simulink subsystem "PvtSubSys_LATC"  (R2020b)
settings: Solver=VariableStepAuto  StartTime=0.0  StopTime=10.0  RelTol=1e-3
values from neighbouring files (symbols this model uses):
  P_Global_CharSpd_ms : value not decoded    [PubParsGlobal.sldd]
  P_Global_SteeringAngleRatio : value not decoded    [PubParsGlobal.sldd]
  P_Global_WheelBase_m : value not decoded    [PubParsGlobal.sldd]
  P_LCS_A0_Limit = 0.25    [LATC.sldd]    (also in LCS_v05.sldd)
  P_LCS_A1_Limit = 0.002    [LATC.sldd]    (also in LCS_v05.sldd)
  P_LCS_communicationTest = 1.0    [LATC.sldd]    (also in LCS_v05.sldd)
  P_LCS_Current_Offset_Test_SW = 0.0    [LATC.sldd]
  P_LCS_Current_Offset_Test_Value = 0.0    [LATC.sldd]
  P_LCS_Curvature_bp : value not decoded    [LATC.sldd]
  P_LCS_CycleTime = 0.4 0.4 0.4 0.4 0.4 0.4 0.4 0.4 0.4 0.6 0.6 0.6 0.6 0.6 0.6 0.6 0.4 0.4 0.4 0.4 0.4 0.4 0.4 0.4 0.4 0.6 0.6 0.6 0.6 0.6 0.6 0.6 0.4 0.4 0.4 0.4 0.4 0.4 0.4 0.4 0.4 0.6 0.6 0.6 0.6 0.6 0.6 0.6 0.4 0.4 0.4 0.4 0.4 0.4 0.4 0.4 0.4 0.6 0.6 0.6 0.6 0.6 0.6 0.6 0.4 0.4 0.4 0.4 0.4 0.4 0.4 0.4 0.4 0.6 0.6 0.6 0.6 0.6 0.6 0.6 0.4 0.4 0.4 0.4 0.4 0.4 0.4 0.4 0.4 0.6 0.6 0.6 0.6 0.6 0.6 0.6 0.4 0.4 0.4 0.4    [LATC.sldd]
  P_LCS_ESS_AngleSlope_Limit = 2.9    [LATC.sldd]    (also in LCS_v05.sldd)
  P_LCS_IN_Offset_Test_SW = 0.0    [LATC.sldd]    (also in LCS_v05.sldd)
  P_LCS_IN_Offset_Test_Value = 0.0    [LATC.sldd]    (also in LCS_v05.sldd)
  P_LCS_LATC_CurOffsetVehicleSpdLimitValue_degs = 7.0    [LATC.sldd]
  P_LCS_LATC_Du_Max = 20.0    [LATC.sldd]
  P_LCS_LATC_ELKAngleSlope_ratio : value not decoded    [LATC.sldd]
  P_LCS_LATC_ELKMaxLatAcc_ms2 : value not decoded    [LATC.sldd]
  P_LCS_LATC_ESSAngleSlope_ratio : value not decoded    [LATC.sldd]
  P_LCS_LATC_ESSMaxLatAcc_ms2 : value not decoded    [LATC.sldd]
  P_LCS_LATC_LCAngleSlope_ratio : value not decoded    [LATC.sldd]
  P_LCS_LATC_LCCancleMaxLatAcc_ms2 : value not decoded    [LATC.sldd]
  P_LCS_LATC_LCEcoAngleSlope_ratio : value not decoded    [LATC.sldd]
  P_LCS_LATC_LCEcoMaxLatAcc_ms2 : value not decoded    [LATC.sldd]
  P_LCS_LATC_LCKAngleSlope_ratio : value not decoded    [LATC.sldd]
  P_LCS_LATC_LCKIEAngleSlope_ratio : value not decoded    [LATC.sldd]
  P_LCS_LATC_LCKIEMaxLatAcc_ms2 : value not decoded    [LATC.sldd]
  P_LCS_LATC_LCKMaxLatAcc_ms2 : value not decoded    [LATC.sldd]
  P_LCS_LATC_LCNormalAngleSlope_ratio : value not decoded    [LATC.sldd]
  P_LCS_LATC_LCNormalMaxLatAcc_ms2 : value not decoded    [LATC.sldd]
  P_LCS_LATC_LCSportAngleSlope_ratio : value not decoded    [LATC.sldd]
  P_LCS_LATC_LCSportMaxLatAcc_ms2 : value not decoded    [LATC.sldd]
  P_LCS_LATC_LKAAngleSlope_ratio : value not decoded    [LATC.sldd]
  P_LCS_LATC_LKAMaxLatAcc_ms2 : value not decoded    [LATC.sldd]
  P_LCS_LATC_MatrixQ1_st = 0.8 0.8 1.2 1.4 1.4 1.4 2.0 2.2 2.2 2.2 2.2 2.2 2.2 2.2 2.2 2.2 0.8 0.8 1.2 1.4 1.4 1.4 2.0 2.2 2.2 2.2 2.2 2.2 2.2 2.2 2.2 2.2 0.8 0.8 1.2 1.4 1.4 1.4 2.0 2.2 2.2 2.2 2.2 2.2 2.2 2.2 2.2 2.2 0.8 0.8 1.2 1.4 1.4 1.4 2.0 2.2 2.2 2.2 2.2 2.2 2.2 2.2 2.2 2.2 0.8 0.8 1.2 1.4 1.4 1.4 2.0 2.2 2.2 2.2 2.2 2.2 2.2 2.2 2.2 2.2 0.8 0.8 1.2 1.4 1.4 1.4 2.0 2.2 2.2 2.2 2.2 2.2 2.2 2.2 2.2 2.2 0.8 0.8 1.2 1.4    [LATC.sldd]
  P_LCS_LATC_MatrixQ3_st = 20.0 20.0 20.0 20.0 20.0 15.0 15.0 15.0 15.0 15.0 15.0 15.0 15.0 13.0 13.0 13.0 20.0 20.0 20.0 20.0 20.0 15.0 15.0 15.0 15.0 15.0 15.0 15.0 15.0 13.0 13.0 13.0 20.0 20.0 20.0 20.0 20.0 15.0 15.0 15.0 15.0 15.0 15.0 15.0 15.0 13.0 13.0 13.0 20.0 20.0 20.0 20.0 20.0 15.0 15.0 15.0 15.0 15.0 15.0 15.0 15.0 13.0 13.0 13.0 20.0 20.0 20.0 20.0 20.0 15.0 15.0 15.0 15.0 15.0 15.0 15.0 15.0 13.0 13.0 13.0    [LATC.sldd]
  P_LCS_LATC_MatrixR_st = 10.0 10.0 10.0 10.0 10.0 10.0 10.0 15.0 15.0 15.0 15.0 15.0 15.0 15.0 15.0 15.0 10.0 10.0 10.0 10.0 10.0 10.0 10.0 15.0 15.0 15.0 15.0 15.0 15.0 15.0 15.0 15.0 10.0 10.0 10.0 10.0 10.0 10.0 10.0 15.0 15.0 15.0 15.0 15.0 15.0 15.0 15.0 15.0 10.0 10.0 10.0 10.0 10.0 10.0 10.0 15.0 15.0 15.0 15.0 15.0 15.0 15.0 15.0 15.0 10.0 10.0 10.0 10.0 10.0 10.0 10.0 15.0 15.0 15.0 15.0 15.0 15.0 15.0 15.0 15.0    [LATC.sldd]
  P_LCS_LATC_Max_LatAcc = 4.0    [LATC.sldd]
  P_LCS_LATC_Max_Phi = 15.0    [LATC.sldd]
  P_LCS_LATC_Max_y = 0.5    [LATC.sldd]
  P_LCS_LATC_MPC_SW = 0.0    [LATC.sldd]
  P_LCS_LATC_PreView_SW = 1.0    [LATC.sldd]
  P_LCS_LATC_SoftConstWeight = 1.0    [LATC.sldd]
  P_LCS_LATC_StateActivAngleSlopeLimit_ratio : value not decoded    [LATC.sldd]
  P_LCS_LATC_StateActiveFlg_TabX_st : value not decoded    [LATC.sldd]
  P_LCS_LATC_StateActiveHoldTime_TabY_st : value not decoded    [LATC.sldd]
  P_LCS_LATC_StateHoldTime_st = 250.0    [LATC.sldd]
  P_LCS_LATC_TarAngleFliterWindowSize = 5.0    [LATC.sldd]
  P_LCS_LATC_TarAngleLP_Time = 0.02    [LATC.sldd]
  P_LCS_LATC_U_Max = 90.0    [LATC.sldd]
  P_LCS_LCK_AngleSlope_Limit = 1.4    [LATC.sldd]
  P_LCS_LineVaildSW = 0.0    [LATC.sldd]
  P_LCS_Lookahead_Distance : value not decoded    [LATC.sldd]
  P_LCS_Lookahead_DistanceFac : value not decoded    [LATC.sldd]
  P_LCS_PLAN_CurvePreView_s = 0.3    [LATC.sldd]
  P_LCS_PLAN_CurvePreview_TabX_m : value not decoded    [LATC.sldd]
  P_LCS_PLAN_CurvePreViewFilterTime_s = 0.1    [LATC.sldd]
  P_LCS_PLAN_ELKAyDtLimit_Tab_ms3 = 1.0 1.0 1.0 1.0 1.0 1.0 1.0 1.0 1.0 1.0 1.0 1.0 1.0 1.0 1.0 1.0 1.0 1.0 1.0 1.0 1.0 1.0 1.0 1.0 1.0 1.0 1.0 1.0 1.0 1.0 1.0 1.0 1.0 1.0 1.0 1.0 1.0 1.0 1.0 1.0 1.0 1.0 1.0 1.0 1.0 1.0 1.0 1.0 1.0 1.0 1.0 1.0 1.0 1.0 1.0 1.0 1.0 1.0 1.0 1.0 1.0 1.0 1.0 1.0 1.0 1.0 1.0 1.0 1.0 1.0 1.0 1.0 1.0 1.0 1.0 1.0 1.0 1.0 1.0 1.0 1.0 1.0 1.0 1.0 1.0 1.0 1.0 1.0 1.0 1.0 1.0 1.0 1.0 1.0 1.0 1.0 1.0 1.0 1.0 1.0    [LATC.sldd]
  P_LCS_PLAN_ESSAyDtLimit_Tab_ms3 = 1.0 1.0 1.0 1.0 1.0 1.0 1.0 1.0 1.0 1.0 1.0 1.0 1.0 1.0 1.0 1.0 1.0 1.0 1.0 1.0 1.0 1.0 1.0 1.0 1.0 1.0 1.0 1.0 1.0 1.0 1.0 1.0 1.0 1.0 1.0 1.0 1.0 1.0 1.0 1.0 1.0 1.0 1.0 1.0 1.0 1.0 1.0 1.0 1.0 1.0 1.0 1.0 1.0 1.0 1.0 1.0 1.0 1.0 1.0 1.0 1.0 1.0 1.0 1.0 1.0 1.0 1.0 1.0 1.0 1.0 1.0 1.0 1.0 1.0 1.0 1.0 1.0 1.0 1.0 1.0 1.0 1.0 1.0 1.0 1.0 1.0 1.0 1.0 1.0 1.0 1.0 1.0 1.0 1.0 1.0 1.0 1.0 1.0 1.0 1.0    [LATC.sldd]
  P_LCS_PLAN_LCCancleAyDtLimit_Tab_ms3 = 1.0 1.0 1.0 1.0 1.0 1.0 1.0 1.0 1.0 1.0 1.0 1.0 1.0 1.0 1.0 1.0 1.0 1.0 1.0 1.0 1.0 1.0 1.0 1.0 1.0 1.0 1.0 1.0 1.0 1.0 1.0 1.0 1.0 1.0 1.0 1.0 1.0 1.0 1.0 1.0 1.0 1.0 1.0 1.0 1.0 1.0 1.0 1.0 1.0 1.0 1.0 1.0 1.0 1.0 1.0 1.0 1.0 1.0 1.0 1.0 1.0 1.0 1.0 1.0 1.0 1.0 1.0 1.0 1.0 1.0 1.0 1.0 1.0 1.0 1.0 1.0 1.0 1.0 1.0 1.0 1.0 1.0 1.0 1.0 1.0 1.0 1.0 1.0 1.0 1.0 1.0 1.0 1.0 1.0 1.0 1.0 1.0 1.0 1.0 1.0    [LATC.sldd]
  P_LCS_PLAN_LCEcoAyDtLimit_Tab_ms3 = 1.0 1.0 1.0 1.0 1.0 1.0 1.0 1.0 1.0 1.0 1.0 1.0 1.0 1.0 1.0 1.0 1.0 1.0 1.0 1.0 1.0 1.0 1.0 1.0 1.0 1.0 1.0 1.0 1.0 1.0 1.0 1.0 1.0 1.0 1.0 1.0 1.0 1.0 1.0 1.0 1.0 1.0 1.0 1.0 1.0 1.0 1.0 1.0 1.0 1.0 1.0 1.0 1.0 1.0 1.0 1.0 1.0 1.0 1.0 1.0 1.0 1.0 1.0 1.0 1.0 1.0 1.0 1.0 1.0 1.0 1.0 1.0 1.0 1.0 1.0 1.0 1.0 1.0 1.0 1.0 1.0 1.0 1.0 1.0 1.0 1.0 1.0 1.0 1.0 1.0 1.0 1.0 1.0 1.0 1.0 1.0 1.0 1.0 1.0 1.0    [LATC.sldd]
  P_LCS_PLAN_LCKAyDtLimit_Tab_ms3 = 1.5 1.5 1.5 1.5 1.5 1.5 1.5 1.5 1.5 1.5 1.5 1.5 1.5 1.5 1.5 1.5 1.5 1.5 1.5 1.5 1.5 1.5 1.5 1.5 1.5 1.5 1.5 1.5 1.5 1.5 1.5 1.5 1.5 1.5 1.5 1.5 1.5 1.5 1.5 1.5 1.5 1.5 1.5 1.5 1.5 1.5 1.5 1.5 1.5 1.5 1.5 1.5 1.5 1.5 1.5 1.5 1.5 1.5 1.5 1.5 1.5 1.5 1.5 1.5 1.5 1.5 1.5 1.5 1.5 1.5 1.5 1.5 1.5 1.5 1.5 1.5 1.5 1.5 1.5 1.5 1.5 1.5 1.5 1.5 1.5 1.5 1.5 1.5 1.5 1.5 1.5 1.5 1.5 1.5 1.5 1.5 1.5 1.5 1.5 1.5    [LATC.sldd]
  P_LCS_PLAN_LCKIEAyDtLimit_Tab_ms3 = 1.0 1.0 1.0 1.0 1.0 1.0 1.0 1.0 1.0 1.0 1.0 1.0 1.0 1.0 1.0 1.0 1.0 1.0 1.0 1.0 1.0 1.0 1.0 1.0 1.0 1.0 1.0 1.0 1.0 1.0 1.0 1.0 1.0 1.0 1.0 1.0 1.0 1.0 1.0 1.0 1.0 1.0 1.0 1.0 1.0 1.0 1.0 1.0 1.0 1.0 1.0 1.0 1.0 1.0 1.0 1.0 1.0 1.0 1.0 1.0 1.0 1.0 1.0 1.0 1.0 1.0 1.0 1.0 1.0 1.0 1.0 1.0 1.0 1.0 1.0 1.0 1.0 1.0 1.0 1.0 1.0 1.0 1.0 1.0 1.0 1.0 1.0 1.0 1.0 1.0 1.0 1.0 1.0 1.0 1.0 1.0 1.0 1.0 1.0 1.0    [LATC.sldd]
  P_LCS_PLAN_LCNormalAyDtLimit_Tab_ms3 = 1.0 1.0 1.0 1.0 1.0 1.0 1.0 1.0 1.0 1.0 1.0 1.0 1.0 1.0 1.0 1.0 1.0 1.0 1.0 1.0 1.0 1.0 1.0 1.0 1.0 1.0 1.0 1.0 1.0 1.0 1.0 1.0 1.0 1.0 1.0 1.0 1.0 1.0 1.0 1.0 1.0 1.0 1.0 1.0 1.0 1.0 1.0 1.0 1.0 1.0 1.0 1.0 1.0 1.0 1.0 1.0 1.0 1.0 1.0 1.0 1.0 1.0 1.0 1.0 1.0 1.0 1.0 1.0 1.0 1.0 1.0 1.0 1.0 1.0 1.0 1.0 1.0 1.0 1.0 1.0 1.0 1.0 1.0 1.0 1.0 1.0 1.0 1.0 1.0 1.0 1.0 1.0 1.0 1.0 1.0 1.0 1.0 1.0 1.0 1.0    [LATC.sldd]
  P_LCS_PLAN_LCSportAyDtLimit_Tab_ms3 = 1.0 1.0 1.0 1.0 1.0 1.0 1.0 1.0 1.0 1.0 1.0 1.0 1.0 1.0 1.0 1.0 1.0 1.0 1.0 1.0 1.0 1.0 1.0 1.0 1.0 1.0 1.0 1.0 1.0 1.0 1.0 1.0 1.0 1.0 1.0 1.0 1.0 1.0 1.0 1.0 1.0 1.0 1.0 1.0 1.0 1.0 1.0 1.0 1.0 1.0 1.0 1.0 1.0 1.0 1.0 1.0 1.0 1.0 1.0 1.0 1.0 1.0 1.0 1.0 1.0 1.0 1.0 1.0 1.0 1.0 1.0 1.0 1.0 1.0 1.0 1.0 1.0 1.0 1.0 1.0 1.0 1.0 1.0 1.0 1.0 1.0 1.0 1.0 1.0 1.0 1.0 1.0 1.0 1.0 1.0 1.0 1.0 1.0 1.0 1.0    [LATC.sldd]
  P_LCS_PLAN_LKAAyDtLimit_Tab_ms3 = 1.0 1.0 1.0 1.0 1.0 1.0 1.0 1.0 1.0 1.0 1.0 1.0 1.0 1.0 1.0 1.0 1.0 1.0 1.0 1.0 1.0 1.0 1.0 1.0 1.0 1.0 1.0 1.0 1.0 1.0 1.0 1.0 1.0 1.0 1.0 1.0 1.0 1.0 1.0 1.0 1.0 1.0 1.0 1.0 1.0 1.0 1.0 1.0 1.0 1.0 1.0 1.0 1.0 1.0 1.0 1.0 1.0 1.0 1.0 1.0 1.0 1.0 1.0 1.0 1.0 1.0 1.0 1.0 1.0 1.0 1.0 1.0 1.0 1.0 1.0 1.0 1.0 1.0 1.0 1.0 1.0 1.0 1.0 1.0 1.0 1.0 1.0 1.0 1.0 1.0 1.0 1.0 1.0 1.0 1.0 1.0 1.0 1.0 1.0 1.0    [LATC.sldd]
  P_LCS_PLAN_MinPlanDis_m : value not decoded    [LATC.sldd]
  P_LCS_PLAN_PreCurMinDisFac_ratio : value not decoded    [LATC.sldd]
  P_LCS_PLAN_PreDisCurve_TabX_m : value not decoded    [LATC.sldd]
  P_LCS_PLAN_StateActiv_AyDtLimit_ms3 : value not decoded    [LATC.sldd]
  P_LCS_PLAN_VehicleSpd_TabX_kph : value not decoded    [LATC.sldd]
  P_LCS_PLAN_VehicleSpd_TabY_Kph : value not decoded    [LATC.sldd]
  P_LCS_Trq_Switch = 0.0    [LATC.sldd]    (also in LCS_v05.sldd)
  P_LCS_VehicleSpd_TabX_Kph : value not decoded    [LATC.sldd]
undefined symbols (not defined in the file or in its folder): HWP_AngCmdReqVal, HWP_AngCmdReqValVld, HWP_FuncTrqCmdReqFlag, HWP_ReqCtrlEPS, HWP_ReqCtrlEPSVld, HWP_TrqOvlCmdReqValue, HWP_WorkReq, HWP_WorkReqVld
libraries: simulink x4, dspbuff3 x2
(part 1 of 8)
settings Model: Creator=GW00184765  LastModifiedBy=GW00216231

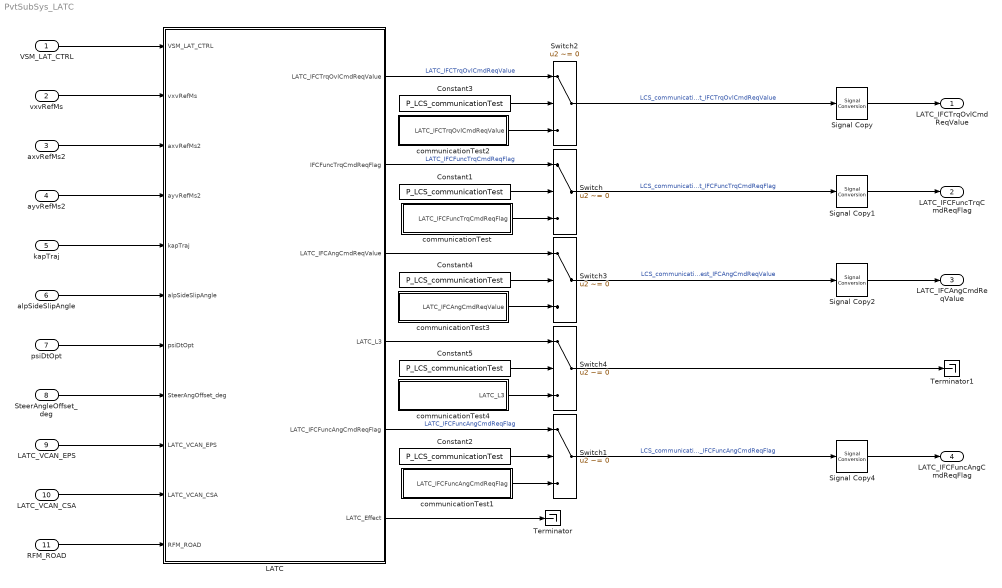
== system PvtSubSys_LATC ==
  VSM_LAT_CTRL : Inport  Description=|  OutDataTypeStr=Bus: VSM_LAT_CTRL_BUS  PortDimensions=1  BusOutputAsStruct=on
      | | 目标线有效性
      | | 目标线多项式系数A3
      | | 目标线多项式系数A2
      | | 目标线多项式系数A1
      | | 目标线多项式系数A0
      | | 功能状态
  vxvRefMs : Inport  Description=ms | 车辆纵向速度  Port=2  OutDataTypeStr=single  PortDimensions=1  BusOutputAsStruct=on
  axvRefMs2 : Inport  Description=ms2 | 车辆纵向加速度  Port=3  OutDataTypeStr=single  PortDimensions=1  BusOutputAsStruct=on
  ayvRefMs2 : Inport  Description=ms2 | 车辆横向加速度  Port=4  OutDataTypeStr=single  PortDimensions=1  BusOutputAsStruct=on
  kapTraj : Inport  Description=m-1 | 自车行驶曲率  Port=5  OutDataTypeStr=single  PortDimensions=1  BusOutputAsStruct=on
  alpSideSlipAngle : Inport  Description=| 车辆后轮侧滑角  Port=6  OutDataTypeStr=single  PortDimensions=1  BusOutputAsStruct=on
  psiDtOpt : Inport  Description=| 自车参考横摆角速度  Port=7  OutDataTypeStr=single  PortDimensions=1  BusOutputAsStruct=on
  SteerAngleOffset_deg : Inport  Description=| 方向盘转角补偿角  Port=8  OutDataTypeStr=single  PortDimensions=1  BusOutputAsStruct=on
  LATC_VCAN_EPS : Inport  Description=|  Port=9  OutDataTypeStr=Bus: VCAN_EPS_MSG_BUS  PortDimensions=1  BusOutputAsStruct=on
      | | 驾驶员手力
      | | EPS叠加力矩
      | | EPS叠加力矩有效性标志位
      | | 角度接口EPS故障状态
      | | 扭矩接口EPS故障状态
      | | EPS故障状态
  LATC_VCAN_CSA : Inport  Description=|  Port=10  OutDataTypeStr=Bus: VCAN_CSA_MSG_BUS  PortDimensions=1  BusOutputAsStruct=on
      | | 方向盘转角方向标志位
      | | 方向盘转角
      | | 方向盘转速方向标志位
      | | 方向盘转速信号
  RFM_ROAD : Inport  Description=m | 车道宽度  Port=11  OutDataTypeStr=Bus: RFM_ROAD_BUS  PortDimensions=1  BusOutputAsStruct=on
  Constant{1..5} (5 alike) : Constant  Description=1  Value=P_LCS_communicationTest
      settings: AttributesFormatString=%<Description>
  LATC : Subsystem
  Signal Copy{,1..2,4} (4 alike) : SignalConversion  OverrideOpt=off
  Switch{,1..4} (5 alike) : Switch  Criteria=u2 ~= 0
  Terminator : Terminator
  Terminator1 : Terminator
  communicationTest : Subsystem
  communicationTest1 : Subsystem
  communicationTest2 : Subsystem
  communicationTest3 : Subsystem
  communicationTest4 : Subsystem
  LATC_IFCTrqOvlCmdReqValue : Outport  Description=| EPS请求扭矩值（EPS扭矩接口）  OutDataTypeStr=single  PortDimensions=1  BusOutputAsStruct=on
  LATC_IFCFuncTrqCmdReqFlag : Outport  Description=| EPS请求扭矩标志位（EPS为扭矩接口）  Port=2  OutDataTypeStr=uint8  PortDimensions=1  BusOutputAsStruct=on
  LATC_IFCAngCmdReqValue : Outport  Description=| EPS请求角度值（EPS为角度接口）  Port=3  OutDataTypeStr=single  PortDimensions=1  BusOutputAsStruct=on
  LATC_IFCFuncAngCmdReqFlag : Outport  Description=| EPS请求扭矩标志位（EPS为角度接口）  Port=4  OutDataTypeStr=uint8  PortDimensions=1  BusOutputAsStruct=on
  wires:
  RFM_ROAD/1 -> LATC/11(RFM_ROAD)
  kapTraj/1 -> LATC/5(kapTraj)
  vxvRefMs/1 -> LATC/2(vxvRefMs)
  alpSideSlipAngle/1 -> LATC/6(alpSideSlipAngle)
  ayvRefMs2/1 -> LATC/4(ayvRefMs2)
  LATC_VCAN_EPS/1 -> LATC/9(LATC_VCAN_EPS)
  LATC/2(IFCFuncTrqCmdReqFlag) -> Switch/1  "LATC_IFCFuncTrqCmdReqFlag"
  psiDtOpt/1 -> LATC/7(psiDtOpt)
  SteerAngleOffset_deg/1 -> LATC/8(SteerAngOffset_deg)
  LATC/4(LATC_L3) -> Switch4/1
  VSM_LAT_CTRL/1 -> LATC/1(VSM_LAT_CTRL)
  axvRefMs2/1 -> LATC/3(axvRefMs2)
  LATC_VCAN_CSA/1 -> LATC/10(LATC_VCAN_CSA)
  LATC/3(LATC_IFCAngCmdReqValue) -> Switch3/1
  LATC/6(LATC_Effect) -> Terminator/1
  Switch2/1 -> Signal Copy/1  "LCS_communicationTest_IFCTrqOvlCmdReqValue"
  Constant3/1 -> Switch2/2
  LATC/1(LATC_IFCTrqOvlCmdReqValue) -> Switch2/1  "LATC_IFCTrqOvlCmdReqValue"
  communicationTest2/1(LATC_IFCTrqOvlCmdReqValue) -> Switch2/3
  Switch/1 -> Signal Copy1/1  "LCS_communicationTest_IFCFuncTrqCmdReqFlag"
  communicationTest/1(LATC_IFCFuncTrqCmdReqFlag) -> Switch/3
  Constant1/1 -> Switch/2
  Constant4/1 -> Switch3/2
  communicationTest3/1(LATC_IFCAngCmdReqValue) -> Switch3/3
  Switch3/1 -> Signal Copy2/1  "LCS_communicationTest_IFCAngCmdReqValue"
  Switch1/1 -> Signal Copy4/1  "LCS_communicationTest_IFCFuncAngCmdReqFlag"
  communicationTest1/1(LATC_IFCFuncAngCmdReqFlag) -> Switch1/3
  Constant2/1 -> Switch1/2
  LATC/5(LATC_IFCFuncAngCmdReqFlag) -> Switch1/1  "LATC_IFCFuncAngCmdReqFlag"
  Constant5/1 -> Switch4/2
  communicationTest4/1(LATC_L3) -> Switch4/3
  Switch4/1 -> Terminator1/1
  Signal Copy/1 -> LATC_IFCTrqOvlCmdReqValue/1
  Signal Copy1/1 -> LATC_IFCFuncTrqCmdReqFlag/1
  Signal Copy2/1 -> LATC_IFCAngCmdReqValue/1
  Signal Copy4/1 -> LATC_IFCFuncAngCmdReqFlag/1

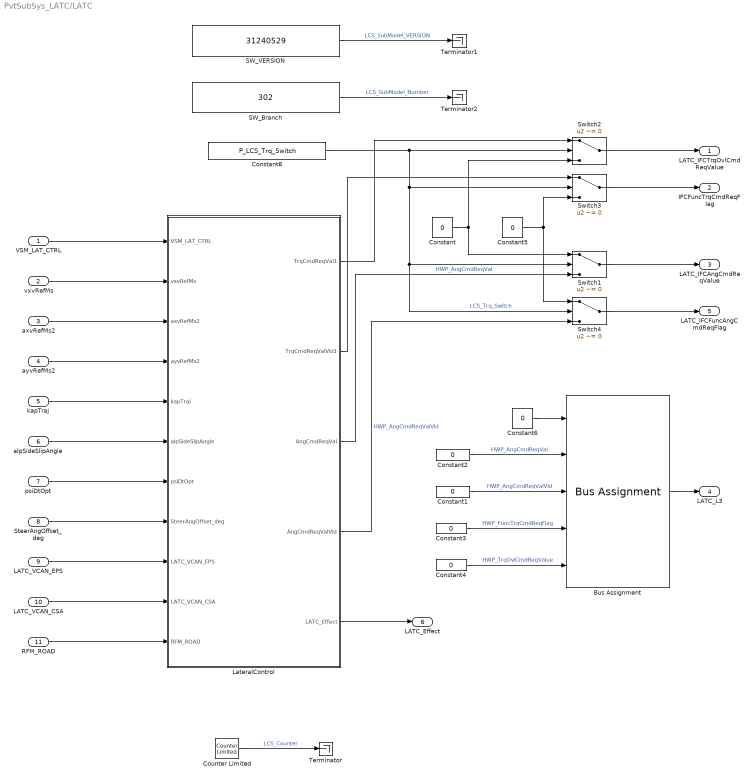
== system PvtSubSys_LATC/LATC ==
  VSM_LAT_CTRL : Inport  Description=|  OutDataTypeStr=Bus: VSM_LAT_CTRL_BUS  PortDimensions=1  Interpolate=off  BusOutputAsStruct=on
      | | 目标线有效性
      | | 目标线多项式系数A3
      | | 目标线多项式系数A2
      | | 目标线多项式系数A1
      | | 目标线多项式系数A0
      | | 功能状态
  vxvRefMs : Inport  Description=ms | 车辆纵向速度  Port=2  OutDataTypeStr=single  PortDimensions=1  Interpolate=off  BusOutputAsStruct=on
  axvRefMs2 : Inport  Description=ms2 | 车辆纵向加速度  Port=3  OutDataTypeStr=single  PortDimensions=1  Interpolate=off  BusOutputAsStruct=on
  ayvRefMs2 : Inport  Description=ms2 | 车辆横向加速度  Port=4  OutDataTypeStr=single  PortDimensions=1  Interpolate=off  BusOutputAsStruct=on
  kapTraj : Inport  Description=m-1 | 自车行驶曲率  Port=5  OutDataTypeStr=single  PortDimensions=1  Interpolate=off  BusOutputAsStruct=on
  alpSideSlipAngle : Inport  Description=| 车辆后轮侧滑角  Port=6  OutDataTypeStr=single  PortDimensions=1  Interpolate=off  BusOutputAsStruct=on
  psiDtOpt : Inport  Description=| 自车参考横摆角速度  Port=7  OutDataTypeStr=single  PortDimensions=1  Interpolate=off  BusOutputAsStruct=on
  SteerAngOffset_deg : Inport  Description=| 方向盘转角补偿角  Port=8  OutDataTypeStr=single  PortDimensions=1  Interpolate=off  BusOutputAsStruct=on
  LATC_VCAN_EPS : Inport  Description=|  Port=9  OutDataTypeStr=Bus: VCAN_EPS_MSG_BUS  PortDimensions=1  BusOutputAsStruct=on
      | | 驾驶员手力
      | | EPS叠加力矩
      | | EPS叠加力矩有效性标志位
      | | 角度接口EPS故障状态
      | | 扭矩接口EPS故障状态
      | | EPS故障状态
  LATC_VCAN_CSA : Inport  Description=|  Port=10  OutDataTypeStr=Bus: VCAN_CSA_MSG_BUS  PortDimensions=1  BusOutputAsStruct=on
      | | 方向盘转角方向标志位
      | | 方向盘转角
      | | 方向盘转速方向标志位
      | | 方向盘转速信号
  RFM_ROAD : Inport  Description=m | 车道宽度  Port=11  OutDataTypeStr=Bus: RFM_ROAD_BUS  PortDimensions=1  BusOutputAsStruct=on
  Bus Assignment : BusAssignment  AssignedSignals=HWP_AngCmdReqVal,HWP_AngCmdReqValVld,HWP_FuncTrqCmdReqFlag,HWP_TrqOvlCmdReqValue
  Constant : Constant  Value=0  OutDataTypeStr=single
  Constant1 : Constant  Value=0  OutDataTypeStr=boolean
  Constant2 : Constant  Value=0  OutDataTypeStr=single
  Constant3 : Constant  Value=0  OutDataTypeStr=uint8
  Constant4 : Constant  Value=0  OutDataTypeStr=single
  Constant5 : Constant  Value=0  OutDataTypeStr=uint8
  Constant6 : Constant  Value=0  OutDataTypeStr=Bus: LATC_L3_BUS
  Constant8 : Constant  Description=0  Value=P_LCS_Trq_Switch  OutDataTypeStr=uint8
      settings: AttributesFormatString=%<Description>
  Counter Limited : simulink/Sources/Counter Limited  uplimit=15  tsamp=-1
  LateralControl : Subsystem
  SW_Branch : Constant  Value=302  OutDataTypeStr=uint32
  SW_VERSION : Constant  Value=31240529  OutDataTypeStr=uint32
  Switch{1..4} (4 alike) : Switch  Criteria=u2 ~= 0
  Terminator : Terminator
  Terminator1 : Terminator
  Terminator2 : Terminator
  LATC_IFCTrqOvlCmdReqValue : Outport  Description=| EPS请求扭矩值（EPS扭矩接口）  OutDataTypeStr=single  PortDimensions=1  BusOutputAsStruct=on
  IFCFuncTrqCmdReqFlag : Outport  Description=| EPS请求扭矩标志位（EPS为扭矩接口）  Port=2  OutDataTypeStr=uint8  PortDimensions=1  BusOutputAsStruct=on
  LATC_IFCAngCmdReqValue : Outport  Description=| EPS请求角度值（EPS为角度接口）  Port=3  OutDataTypeStr=single  PortDimensions=1  BusOutputAsStruct=on
  LATC_L3 : Outport  Description=|  Port=4  OutDataTypeStr=Bus: LATC_L3_BUS
      | | HWP角度请求值（EPS为角度接口）
      | | HWP角度请求值标志位（EPS为角度接口）
      | | HWP请求EPS控制标志位
      | | HWP请求EPS控制标志位有效性
      | | HWP工作请求标志位
      | | HWP工作请求标志位有效性
      | | HWP请求扭矩标志位（EPS为扭矩接口）
      | | HWP请求扭矩值（EPS为扭矩接口）
  LATC_IFCFuncAngCmdReqFlag : Outport  Description=| EPS请求扭矩标志位（EPS为角度接口）  Port=5  OutDataTypeStr=uint8  PortDimensions=1  BusOutputAsStruct=on
  LATC_Effect : Outport  Port=6  OutDataTypeStr=single
  wires:
  Bus Assignment/1 -> LATC_L3/1
  Constant6/1 -> Bus Assignment/1
  LateralControl/2(TrqCmdReqValVld1) -> Switch3/1
  LateralControl/1(TrqCmdReqVal1) -> Switch2/1
  LateralControl/5(LATC_Effect) -> LATC_Effect/1
  Counter Limited/1 -> Terminator/1  "LCS_Counter"
  LATC_VCAN_CSA/1 -> LateralControl/10(LATC_VCAN_CSA)
  VSM_LAT_CTRL/1 -> LateralControl/1(VSM_LAT_CTRL)
  psiDtOpt/1 -> LateralControl/7(psiDtOpt)
  ayvRefMs2/1 -> LateralControl/4(ayvRefMs2)
  RFM_ROAD/1 -> LateralControl/11(RFM_ROAD)
  SteerAngOffset_deg/1 -> LateralControl/8(SteerAngOffset_deg)
  vxvRefMs/1 -> LateralControl/2(vxvRefMs)
  kapTraj/1 -> LateralControl/5(kapTraj)
  alpSideSlipAngle/1 -> LateralControl/6(alpSideSlipAngle)
  axvRefMs2/1 -> LateralControl/3(axvRefMs2)
  LATC_VCAN_EPS/1 -> LateralControl/9(LATC_VCAN_EPS)
  Constant2/1 -> Bus Assignment/2  "HWP_AngCmdReqVal"
  Constant3/1 -> Bus Assignment/4  "HWP_FuncTrqCmdReqFlag"
  Constant4/1 -> Bus Assignment/5  "HWP_TrqOvlCmdReqValue"
  Constant1/1 -> Bus Assignment/3  "HWP_AngCmdReqValVld"
  SW_VERSION/1 -> Terminator1/1  "LCS_SubModel_VERSION"
  SW_Branch/1 -> Terminator2/1  "LCS_SubModel_Number"
  Constant/1 -> Switch2/3, Switch1/1
  Constant5/1 -> Switch4/1, Switch3/3
  Constant8/1 -> Switch3/2, Switch4/2, Switch1/2, Switch2/2  "LCS_Trq_Switch"
  Switch2/1 -> LATC_IFCTrqOvlCmdReqValue/1
  Switch1/1 -> LATC_IFCAngCmdReqValue/1
  LateralControl/3(AngCmdReqVal) -> Switch1/3  "HWP_AngCmdReqVal"
  Switch3/1 -> IFCFuncTrqCmdReqFlag/1
  Switch4/1 -> LATC_IFCFuncAngCmdReqFlag/1
  LateralControl/4(AngCmdReqValVld) -> Switch4/3  "HWP_AngCmdReqValVld"

== system PvtSubSys_LATC/communicationTest ==
  MATLAB Function19 : MATLAB Function  TreatAsAtomicUnit=on
  Unit Delay8 : UnitDelay  InitialCondition=uint8(0)  SampleTime=-1  HasFrameUpgradeWarning=on
  Unit Delay9 : UnitDelay  InitialCondition=uint8(0)  SampleTime=-1  HasFrameUpgradeWarning=on
  LATC_IFCFuncTrqCmdReqFlag : Outport  Description=| EPS请求扭矩值（EPS为扭矩接口）  OutDataTypeStr=uint8  PortDimensions=1  BusOutputAsStruct=on
  wires:
  Unit Delay9/1 -> MATLAB Function19/2(countk1)
  MATLAB Function19/2(count) -> Unit Delay9/1
  Unit Delay8/1 -> MATLAB Function19/1(uint8outK1)
  MATLAB Function19/1(uint8out) -> LATC_IFCFuncTrqCmdReqFlag/1, Unit Delay8/1

== system PvtSubSys_LATC/communicationTest1 ==
  MATLAB Function19 : MATLAB Function  TreatAsAtomicUnit=on
  Unit Delay8 : UnitDelay  InitialCondition=uint8(0)  SampleTime=-1  HasFrameUpgradeWarning=on
  Unit Delay9 : UnitDelay  InitialCondition=uint8(0)  SampleTime=-1  HasFrameUpgradeWarning=on
  LATC_IFCFuncAngCmdReqFlag : Outport  Description=| EPS请求扭矩标志位（EPS为角度接口）  OutDataTypeStr=uint8  PortDimensions=1  BusOutputAsStruct=on
  wires:
  MATLAB Function19/1(uint8out) -> LATC_IFCFuncAngCmdReqFlag/1, Unit Delay8/1
  Unit Delay8/1 -> MATLAB Function19/1(uint8outK1)
  MATLAB Function19/2(count) -> Unit Delay9/1
  Unit Delay9/1 -> MATLAB Function19/2(countk1)

== system PvtSubSys_LATC/communicationTest2 ==
  Constant16 : Constant  Value=-10.23  OutDataTypeStr=single
  Constant17 : Constant  Value=0.01  OutDataTypeStr=single
  Constant18 : Constant  Value=10.24  OutDataTypeStr=single
  MATLAB Function7 : MATLAB Function  TreatAsAtomicUnit=on
  Unit Delay19 : UnitDelay  InitialCondition=uint8(0)  SampleTime=-1  HasFrameUpgradeWarning=on
  Unit Delay20 : UnitDelay  InitialCondition=single(-10.23)  SampleTime=-1  HasFrameUpgradeWarning=on
  LATC_IFCTrqOvlCmdReqValue : Outport  Description=Nm | EPS请求扭矩值（EPS为扭矩接口）  OutDataTypeStr=single  PortDimensions=1  BusOutputAsStruct=on
  wires:
  Unit Delay19/1 -> MATLAB Function7/5(countk1)
  Constant17/1 -> MATLAB Function7/1(factor)
  Constant18/1 -> MATLAB Function7/3(singlemax)
  MATLAB Function7/1(singleout) -> LATC_IFCTrqOvlCmdReqValue/1, Unit Delay20/1
  Unit Delay20/1 -> MATLAB Function7/4(singleoutK1)
  Constant16/1 -> MATLAB Function7/2(singlemin)
  MATLAB Function7/2(count) -> Unit Delay19/1

== system PvtSubSys_LATC/communicationTest3 ==
  Constant16 : Constant  Value=-780  OutDataTypeStr=single
  Constant17 : Constant  Value=0.1  OutDataTypeStr=single
  Constant18 : Constant  Value=780  OutDataTypeStr=single
  MATLAB Function7 : MATLAB Function  TreatAsAtomicUnit=on
  Unit Delay19 : UnitDelay  InitialCondition=uint8(0)  SampleTime=-1  HasFrameUpgradeWarning=on
  Unit Delay20 : UnitDelay  InitialCondition=single(0)  SampleTime=-1  HasFrameUpgradeWarning=on
  LATC_IFCAngCmdReqValue : Outport  Description=deg | EPS请求角度值（EPS为角度接口）  OutDataTypeStr=single  PortDimensions=1  BusOutputAsStruct=on
  wires:
  MATLAB Function7/2(count) -> Unit Delay19/1
  Constant16/1 -> MATLAB Function7/2(singlemin)
  Unit Delay20/1 -> MATLAB Function7/4(singleoutK1)
  MATLAB Function7/1(singleout) -> LATC_IFCAngCmdReqValue/1, Unit Delay20/1
  Constant18/1 -> MATLAB Function7/3(singlemax)
  Constant17/1 -> MATLAB Function7/1(factor)
  Unit Delay19/1 -> MATLAB Function7/5(countk1)

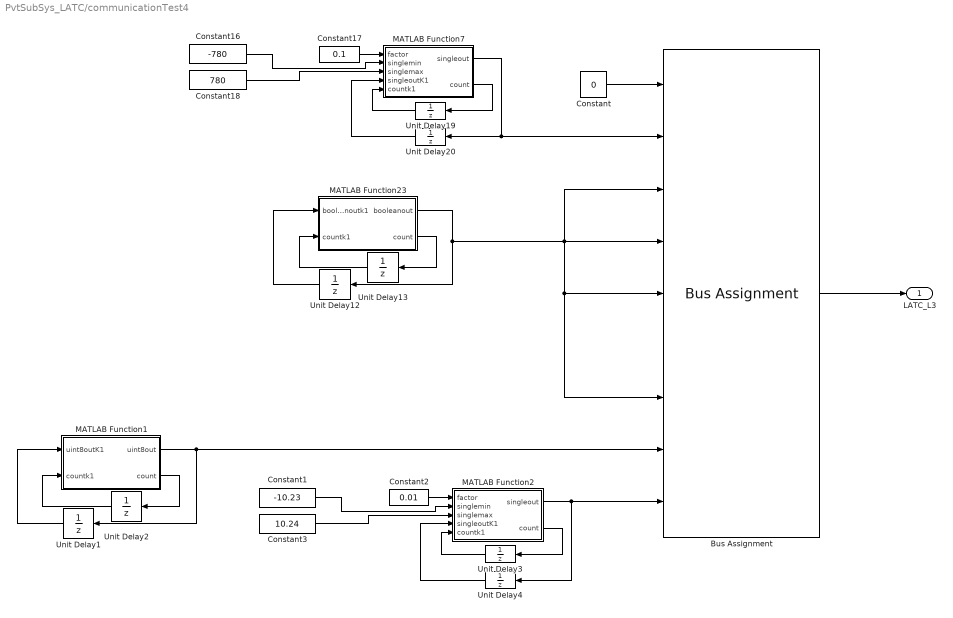
== system PvtSubSys_LATC/communicationTest4 ==
  Bus Assignment : BusAssignment  AssignedSignals=HWP_AngCmdReqVal,HWP_AngCmdReqValVld,HWP_ReqCtrlEPS,HWP_ReqCtrlEPSVld,HWP_WorkReq,HWP_WorkReqVld,HWP_FuncTrqCmdReqFlag,HWP_TrqOvlCmdReqValue
  Constant : Constant  Value=0  OutDataTypeStr=Bus: LATC_L3_BUS
  Constant1 : Constant  Value=-10.23  OutDataTypeStr=single
  Constant16 : Constant  Value=-780  OutDataTypeStr=single
  Constant17 : Constant  Value=0.1  OutDataTypeStr=single
  Constant18 : Constant  Value=780  OutDataTypeStr=single
  Constant2 : Constant  Value=0.01  OutDataTypeStr=single
  Constant3 : Constant  Value=10.24  OutDataTypeStr=single
  MATLAB Function1 : MATLAB Function  TreatAsAtomicUnit=on
  MATLAB Function2 : MATLAB Function  TreatAsAtomicUnit=on
  MATLAB Function23 : MATLAB Function  TreatAsAtomicUnit=on
  MATLAB Function7 : MATLAB Function  TreatAsAtomicUnit=on
  Unit Delay{1..3,13,19} (5 alike) : UnitDelay  InitialCondition=uint8(0)  SampleTime=-1  HasFrameUpgradeWarning=on
  Unit Delay12 : UnitDelay  InitialCondition=false  SampleTime=-1  HasFrameUpgradeWarning=on
  Unit Delay20 : UnitDelay  InitialCondition=single(0)  SampleTime=-1  HasFrameUpgradeWarning=on
  Unit Delay4 : UnitDelay  InitialCondition=single(-10.23)  SampleTime=-1  HasFrameUpgradeWarning=on
  LATC_L3 : Outport  Description=|  OutDataTypeStr=Bus: LATC_L3_BUS  PortDimensions=1  BusOutputAsStruct=on
      | | HWP角度请求值（EPS为角度接口）
      | | HWP角度请求值标志位（EPS为角度接口）
      | | HWP请求EPS控制标志位
      | | HWP请求EPS控制标志位有效性
      | | HWP工作请求标志位
      | | HWP工作请求标志位有效性
      | | HWP请求扭矩标志位（EPS为扭矩接口）
      | | HWP请求扭矩值（EPS为扭矩接口）
  wires:
  MATLAB Function23/1(booleanout) -> Bus Assignment/4, Bus Assignment/5, Bus Assignment/7, Bus Assignment/3, Unit Delay12/1
  Unit Delay12/1 -> MATLAB Function23/1(booleanoutk1)
  MATLAB Function23/2(count) -> Unit Delay13/1
  Unit Delay13/1 -> MATLAB Function23/2(countk1)
  Constant2/1 -> MATLAB Function2/1(factor)
  MATLAB Function2/2(count) -> Unit Delay3/1
  Constant1/1 -> MATLAB Function2/2(singlemin)
  Unit Delay3/1 -> MATLAB Function2/5(countk1)
  MATLAB Function2/1(singleout) -> Unit Delay4/1, Bus Assignment/9
  Unit Delay4/1 -> MATLAB Function2/4(singleoutK1)
  Constant3/1 -> MATLAB Function2/3(singlemax)
  Unit Delay1/1 -> MATLAB Function1/1(uint8outK1)
  MATLAB Function1/1(uint8out) -> Unit Delay1/1, Bus Assignment/8
  MATLAB Function1/2(count) -> Unit Delay2/1
  Unit Delay2/1 -> MATLAB Function1/2(countk1)
  Bus Assignment/1 -> LATC_L3/1
  Constant/1 -> Bus Assignment/1
  Unit Delay19/1 -> MATLAB Function7/5(countk1)
  Constant17/1 -> MATLAB Function7/1(factor)
  Constant18/1 -> MATLAB Function7/3(singlemax)
  MATLAB Function7/1(singleout) -> Bus Assignment/2, Unit Delay20/1
  Unit Delay20/1 -> MATLAB Function7/4(singleoutK1)
  Constant16/1 -> MATLAB Function7/2(singlemin)
  MATLAB Function7/2(count) -> Unit Delay19/1
